simulink model "isothermalCSTR"  (R2017a)
settings: Solver=VariableStepAuto  StartTime=0.0  StopTime=30  RelTol=1e-3
values from neighbouring files (symbols this model uses):
  cAf = 10    [iso_cstr_main.m]    (also in iso_model.m)
  K1 = 5/6    (= 0.833333333333)    [iso_cstr_main.m]    (also in iso_model.m)
  K2 = 20/3    (= 6.66666666667)    [iso_cstr_main.m]    (also in iso_model.m = 1.66666666667)
  K3 = 1/6    (= 0.166666666667)    [iso_cstr_main.m]    (also in iso_model.m)
  V = 1    [iso_cstr_main.m]    (also in iso_model.m)
  y0 = [cA_e cB_e cC_e cD_e]    [iso_cstr_main.m]
settings Model: Creator=minhotmog  LastModifiedBy=minhotmog

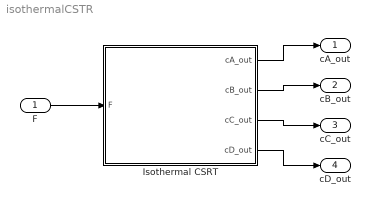
== system isothermalCSTR ==
  F : Inport
  Isothermal CSRT : Subsystem
  cA_out : Outport
  cB_out : Outport  Port=2
  cC_out : Outport  Port=3
  cD_out : Outport  Port=4
  wires:
  Isothermal CSRT/3(cC_out) -> cC_out/1
  Isothermal CSRT/1(cA_out) -> cA_out/1
  Isothermal CSRT/4(cD_out) -> cD_out/1
  Isothermal CSRT/2(cB_out) -> cB_out/1
  F/1 -> Isothermal CSRT/1(F)

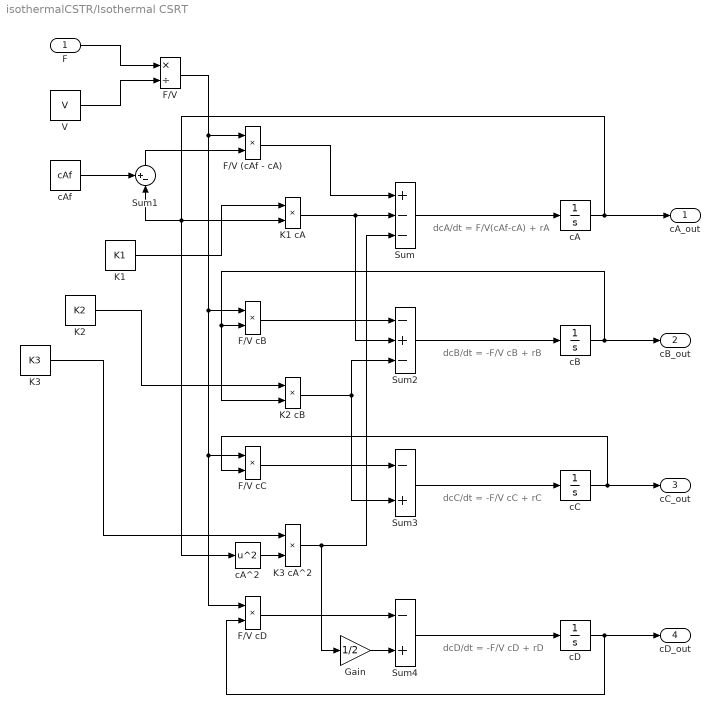
== system isothermalCSTR/Isothermal CSRT ==
  note: dcA/dt = F/V(cAf-cA) + rA
  note: dcB/dt = -F/V cB + rB
  note: dcC/dt = -F/V cC + rC
  note: dcD/dt = -F/V cD + rD
  F : Inport
  F/V : Product  Inputs=*/
  F/V (cAf - cA) : Product  Inputs=**
  F/V cB : Product  Inputs=**
  F/V cC : Product  Inputs=**
  F/V cD : Product  Inputs=**
  Gain : Gain  Gain=1/2
  K1 : Constant  Value=K1
  K1 cA : Product
  K2 : Constant  Value=K2
  K2 cB : Product
  K3 : Constant  Value=K3
  K3 cA^2 : Product
  Sum : Sum  Inputs=+--
  Sum1 : Sum  Inputs=+-|
  Sum2 : Sum  Inputs=-+-
  Sum3 : Sum  Inputs=-+
  Sum4 : Sum  Inputs=-+
  V : Constant  Value=V
  cA : Integrator  InitialCondition=y0(1)
  cA^2 : Fcn  Expr=u^2
  cAf : Constant  Value=cAf
  cB : Integrator  InitialCondition=y0(2)
  cC : Integrator  InitialCondition=y0(3)
  cD : Integrator  InitialCondition=y0(4)
  cA_out : Outport
  cB_out : Outport  Port=2
  cC_out : Outport  Port=3
  cD_out : Outport  Port=4
  wires:
  K2/1 -> K2 cB/1
  F/V (cAf - cA)/1 -> Sum/1
  K1/1 -> K1 cA/1
  cD/1 -> cD_out/1, F/V cD/2
  Sum2/1 -> cB/1
  Sum4/1 -> cD/1
  K3 cA^2/1 -> Gain/1, Sum/3
  V/1 -> F/V/2
  F/V cB/1 -> Sum2/1
  cC/1 -> cC_out/1, F/V cC/2
  F/V cC/1 -> Sum3/1
  K2 cB/1 -> Sum3/2, Sum2/3
  Sum1/1 -> F/V (cAf - cA)/2
  Sum3/1 -> cC/1
  K3/1 -> K3 cA^2/1
  Gain/1 -> Sum4/2
  cB/1 -> cB_out/1, F/V cB/2, K2 cB/2
  F/V/1 -> F/V (cAf - cA)/1, F/V cB/1, F/V cD/1, F/V cC/1
  cAf/1 -> Sum1/1
  F/1 -> F/V/1
  F/V cD/1 -> Sum4/1
  K1 cA/1 -> Sum2/2, Sum/2
  cA/1 -> cA_out/1, Sum1/2, K1 cA/2, cA^2/1
  Sum/1 -> cA/1
  cA^2/1 -> K3 cA^2/2
